simulink model "process_sensors"  (R2025b)
settings: configuration reference "MCConfiguration" (kept outside this file)
undefined symbols (not defined in the file): motorsensors
libraries: dspsigops x2, mcbhdlpositiondecoderlib x1
settings Model: DataDictionary=embeddedBoard_common.sldd  Creator=rpumpo  LastModifiedBy=mfussi
settings ConfigSetRef: SourceName=MCConfiguration

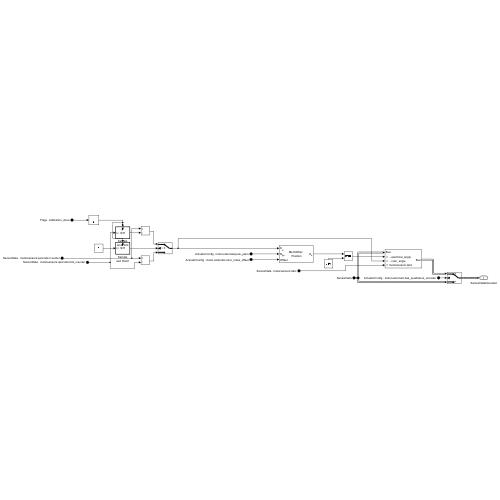
[thumbnail: Simulink's stored preview of the top-level diagram]
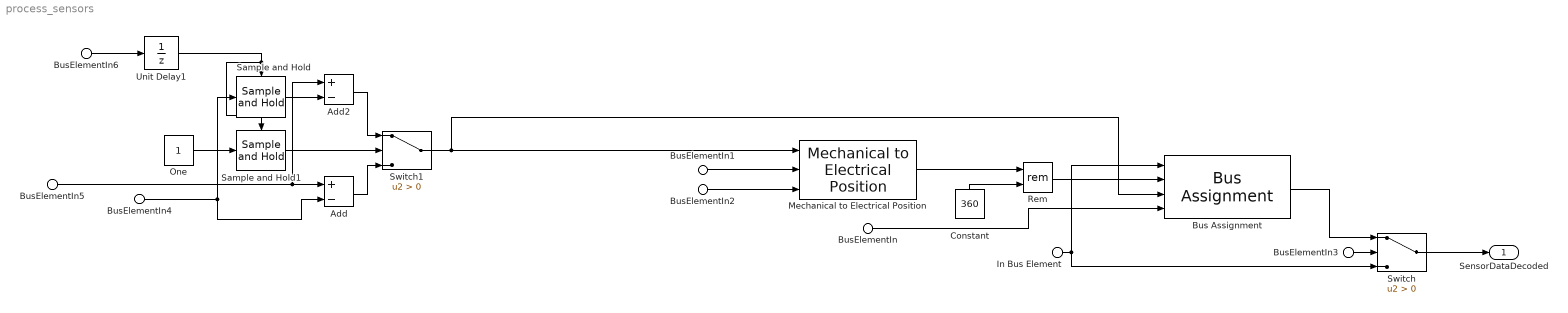
== system process_sensors ==
  BusElementIn3 : Inport  PortName=ActuatorConfig  Element=motor.externals.has_quadrature_encoder
  BusElementIn1 : Inport  PortName=ActuatorConfig  Element=motor.externals.pole_pairs
  BusElementIn2 : Inport  PortName=ActuatorConfig  Element=motor.externals.rotor_index_offset
  BusElementIn6 : Inport  Port=2  PortName=Flags  Element=calibration_done
  In Bus Element : Inport  Port=3  PortName=SensorData
  BusElementIn5 : Inport  Description=Counter of the QENC  Port=3  PortName=SensorData  Element=motorsensors.qencoder.counter
  BusElementIn4 : Inport  Description=Last QENC count where the index has been detected  Port=3  PortName=SensorData  Element=motorsensors.qencoder.Idx_counter
  BusElementIn : Inport  Port=3  PortName=SensorData  Element=motorsensors.Iabc
  Add : Sum  Inputs=+-
  Add2 : Sum  Inputs=+-
  Bus Assignment : BusAssignment  AssignedSignals=motorsensors.electrical_angle,motorsensors.qencoder.rotor_angle,motorsensors.Iabc
  Constant : Constant  Value=360  OutDataTypeStr=single
  Mechanical to Electrical Position : mcbhdlpositiondecoderlib/Mechanical to Electrical Position  PolePairsInputType=Input port  NrPP=4  selectedRange=Degrees  MechOfstInputType=Input port  mechOffsetIn=0  maxAngleIn=360  InputDataType=single  VariantSelect=floating-point
      settings: LibrarySourceBlock=mcbhdllib/Sensor Decoders/Mechanical to Electrical Position
  One : Constant  OutDataTypeStr=Inherit: Inherit via back propagation
  Rem : Math  Operator=rem
  Sample and Hold : dspsigops/Sample and Hold  trig=Rising edge  initCond=0  latchinput=off
  Sample and Hold1 : dspsigops/Sample and Hold  trig=Rising edge  initCond=0  latchinput=off
  Switch : Switch  Criteria=u2 > Threshold  SaturateOnIntegerOverflow=off  InputSameDT=off
  Switch1 : Switch  Criteria=u2 > Threshold  SaturateOnIntegerOverflow=off  InputSameDT=off
  Unit Delay1 : UnitDelay  SampleTime=-1  HasFrameUpgradeWarning=on
  SensorDataDecoded : Outport  OutDataTypeStr=Bus: SensorsData  BusOutputAsStruct=on
  wires:
  BusElementIn3/1 -> Switch/2
  Constant/1 -> Rem/2
  BusElementIn5/1 -> Add2/1, Add/1
  Add2/1 -> Switch1/1
  In Bus Element/1 -> Bus Assignment/1, Switch/3
  Unit Delay1/1 -> Sample and Hold1/Trigger, Sample and Hold/Trigger
  Switch/1 -> SensorDataDecoded/1
  Sample and Hold1/1 -> Switch1/2
  Rem/1 -> Bus Assignment/2
  BusElementIn2/1 -> Mechanical to Electrical Position/3
  Switch1/1 -> Mechanical to Electrical Position/1, Bus Assignment/3
  Add/1 -> Switch1/3
  BusElementIn1/1 -> Mechanical to Electrical Position/2
  One/1 -> Sample and Hold1/1
  Sample and Hold/1 -> Add2/2
  Bus Assignment/1 -> Switch/1
  BusElementIn4/1 -> Sample and Hold/1, Add/2
  Mechanical to Electrical Position/1 -> Rem/1
  BusElementIn6/1 -> Unit Delay1/1
  BusElementIn/1 -> Bus Assignment/4
